simulink model "problem4_simulink_"  (R2021a)
settings: Solver=VariableStepAuto  StartTime=0.0  StopTime=100  RelTol=1e-3
values from neighbouring files (symbols this model uses):
  a4 = init + (last+init)*rand(N,1)    [problem4_code_.m]
  a_hat_ic = init + (last+init)*rand(N,1)    [problem4_code_.m]
  alpha4 = 0.1    [problem4_code_.m]
  beta4 = 0.1    [problem4_code_.m]
  c4 = init + (last+init)*rand(N,1)    [problem4_code_.m]
  g4 = 9.8    [problem4_code_.m]
  gamma4 = diag(gamma)    [problem4_code_.m]
  gamma_a4 = 0.1    [problem4_code_.m]
  k4 = init + (last+init)*rand(N,1)    [problem4_code_.m]
  m4 = init + (last+init)*rand(N,1)    [problem4_code_.m]
  phi4 = init + (last+init)*rand(N,1)    [problem4_code_.m]
  s4 = 0.1    [problem4_code_.m]
  theta = [m4, c4, k4]    [problem4_code_.m]
  theta_hat_ic = [init + (last+init)*rand(N,1), init + (last+init)*rand(N,1), init + (last+init)*rand(N,1)]    [problem4_code_.m]
  u_ic4 = 0    [problem4_code_.m]
  x_ic4 = init + (last+init)*randn(N,1)    [problem4_code_.m]
  xd4 = init + (last+init)*randn(N,1)    [problem4_code_.m]
  xdot_ic4 = 0    [problem4_code_.m]
settings Model: Creator=kaush  LastModifiedBy=kaush
settings DebuggingCC: UnderSpecifiedDimensionMsg=warning

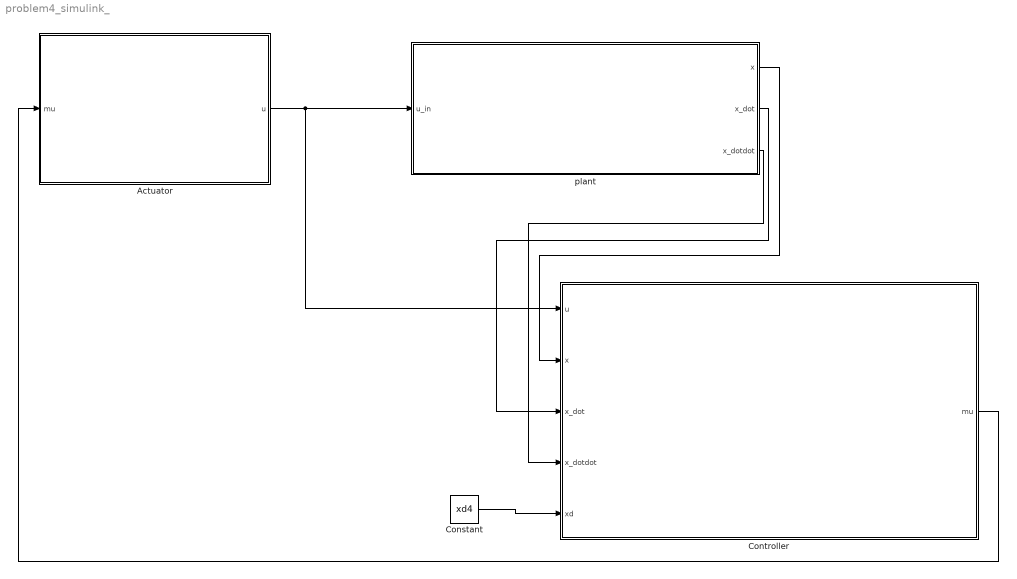
== system problem4_simulink_ ==
  Actuator : Subsystem
  Constant : Constant  Value=xd4
  Controller : Subsystem
  plant : Subsystem
  wires:
  Actuator/1(u) -> Controller/1(u), plant/1(u_in)
  plant/1(x) -> Controller/2(x)
  plant/2(x_dot) -> Controller/3(x_dot)
  plant/3(x_dotdot) -> Controller/4(x_dotdot)
  Constant/1 -> Controller/5(xd)
  Controller/1(mu) -> Actuator/1(mu)

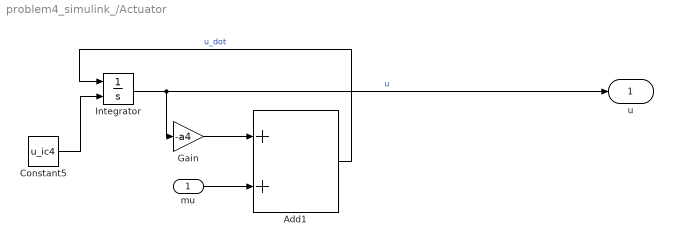
== system problem4_simulink_/Actuator ==
  mu : Inport
  Add1 : Sum
  Constant5 : Constant  Value=u_ic4
  Gain : Gain  Gain=-a4
  Integrator : Integrator  InitialConditionSource=external
  u : Outport
  wires:
  Add1/1 -> Integrator/1  "u_dot"
  Integrator/1 -> u/1, Gain/1  "u"
  Gain/1 -> Add1/1
  mu/1 -> Add1/2
  Constant5/1 -> Integrator/2

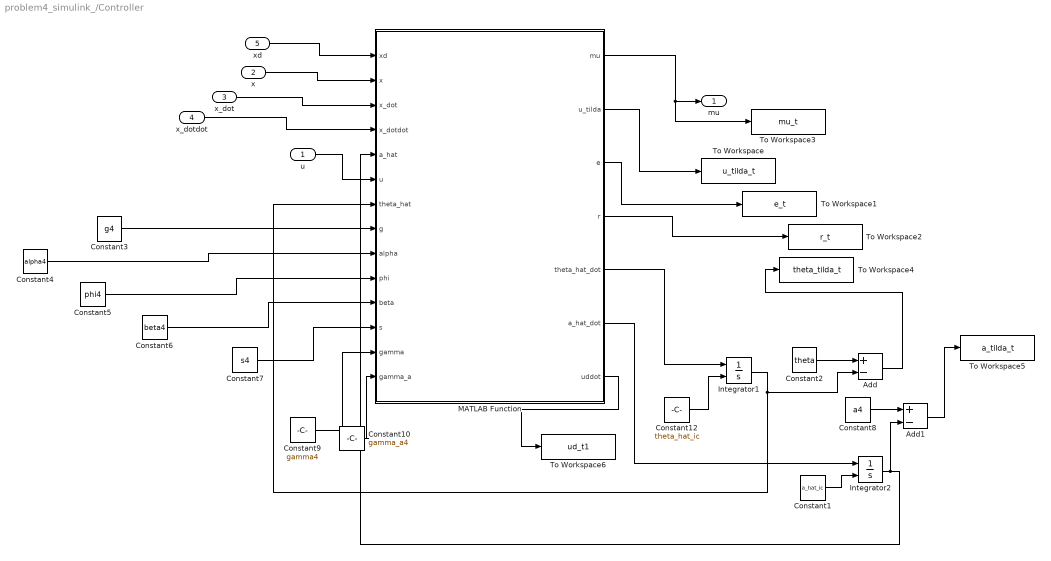
== system problem4_simulink_/Controller ==
  u : Inport
  x : Inport  Port=2
  x_dot : Inport  Port=3
  x_dotdot : Inport  Port=4
  xd : Inport  Port=5
  Add : Sum  Inputs=+-
  Add1 : Sum  Inputs=+-
  Constant1 : Constant  Value=a_hat_ic
  Constant10 : Constant  Value=gamma_a4
  Constant12 : Constant  Value=theta_hat_ic
  Constant2 : Constant  Value=theta
  Constant3 : Constant  Value=g4
  Constant4 : Constant  Value=alpha4
  Constant5 : Constant  Value=phi4
  Constant6 : Constant  Value=beta4
  Constant7 : Constant  Value=s4
  Constant8 : Constant  Value=a4
  Constant9 : Constant  Value=gamma4
  Integrator1 : Integrator  InitialConditionSource=external
  Integrator2 : Integrator  InitialConditionSource=external
  MATLAB Function : MATLAB Function  TreatAsAtomicUnit=on
  To Workspace : ToWorkspace  VariableName=u_tilda_t  SaveFormat=Timeseries  SampleTime=-1
  To Workspace1 : ToWorkspace  VariableName=e_t  SaveFormat=Timeseries  SampleTime=-1
  To Workspace2 : ToWorkspace  VariableName=r_t  SaveFormat=Timeseries  SampleTime=-1
  To Workspace3 : ToWorkspace  VariableName=mu_t  SaveFormat=Timeseries  SampleTime=-1
  To Workspace4 : ToWorkspace  VariableName=theta_tilda_t  SaveFormat=Timeseries  SampleTime=-1
  To Workspace5 : ToWorkspace  VariableName=a_tilda_t  SaveFormat=Timeseries  SampleTime=-1
  To Workspace6 : ToWorkspace  VariableName=ud_t1  SaveFormat=Timeseries  SampleTime=-1
  mu : Outport
  wires:
  x/1 -> MATLAB Function/2(x)
  Constant7/1 -> MATLAB Function/12(s)
  Constant3/1 -> MATLAB Function/8(g)
  Constant6/1 -> MATLAB Function/11(beta)
  Constant4/1 -> MATLAB Function/9(alpha)
  u/1 -> MATLAB Function/6(u)
  x_dotdot/1 -> MATLAB Function/4(x_dotdot)
  xd/1 -> MATLAB Function/1(xd)
  MATLAB Function/3(e) -> To Workspace1/1
  MATLAB Function/2(u_tilda) -> To Workspace/1
  Constant5/1 -> MATLAB Function/10(phi)
  x_dot/1 -> MATLAB Function/3(x_dot)
  MATLAB Function/1(mu) -> To Workspace3/1, mu/1
  MATLAB Function/4(r) -> To Workspace2/1
  Add/1 -> To Workspace4/1
  Add1/1 -> To Workspace5/1
  Constant9/1 -> MATLAB Function/13(gamma)
  Constant10/1 -> MATLAB Function/14(gamma_a)
  Constant12/1 -> Integrator1/2
  MATLAB Function/5(theta_hat_dot) -> Integrator1/1
  Integrator1/1 -> MATLAB Function/7(theta_hat), Add/2
  Constant1/1 -> Integrator2/2
  MATLAB Function/6(a_hat_dot) -> Integrator2/1
  Integrator2/1 -> Add1/2, MATLAB Function/5(a_hat)
  Constant2/1 -> Add/1
  Constant8/1 -> Add1/1
  MATLAB Function/7(uddot) -> To Workspace6/1

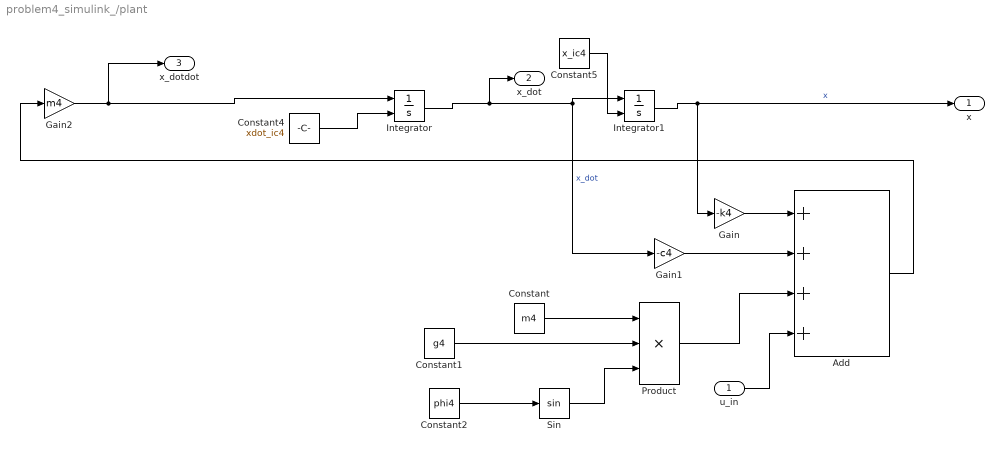
== system problem4_simulink_/plant ==
  u_in : Inport
  Add : Sum  Inputs=++++
  Constant : Constant  Value=m4
  Constant1 : Constant  Value=g4
  Constant2 : Constant  Value=phi4
  Constant4 : Constant  Value=xdot_ic4
  Constant5 : Constant  Value=x_ic4
  Gain : Gain  Gain=-k4
  Gain1 : Gain  Gain=-c4
  Gain2 : Gain  Gain=m4
  Integrator : Integrator  InitialConditionSource=external
  Integrator1 : Integrator  InitialConditionSource=external
  Product : Product  Inputs=3
  Sin : Trigonometry
  x : Outport
  x_dot : Outport  Port=2
  x_dotdot : Outport  Port=3
  wires:
  Constant1/1 -> Product/2
  Product/1 -> Add/3
  Sin/1 -> Product/3
  Constant4/1 -> Integrator/2
  Constant5/1 -> Integrator1/2
  u_in/1 -> Add/4
  Gain2/1 -> Integrator/1, x_dotdot/1
  Integrator/1 -> x_dot/1, Integrator1/1, Gain1/1  "x_dot"
  Gain/1 -> Add/1
  Constant/1 -> Product/1
  Gain1/1 -> Add/2
  Add/1 -> Gain2/1
  Integrator1/1 -> x/1, Gain/1  "x"
  Constant2/1 -> Sin/1

== matlab function problem4_simulink_/Controller/MATLAB Function ==
  data: xd input; mu output; x input; x_dot input; x_dotdot input; a_hat input; u input; theta_hat input; g input; alpha input; phi input; beta input; s input; u_tilda output; e output; r output; gamma input; gamma_a input; theta_hat_dot output; a_hat_dot output; uddot output
function [mu,u_tilda,e,r, theta_hat_dot, a_hat_dot,uddot] = fcn(xd,x,x_dot,x_dotdot, a_hat, u, theta_hat, g, alpha, phi, beta, s, gamma, gamma_a)
e = xd - x;
e_dot = -x_dot;
e_dotdot = -x_dotdot;
r = e_dot + alpha*e;
r_dot = e_dotdot + alpha*e_dot;
Y = [-g*sin(phi)+alpha*e_dot, x_dot, x];
Y_dot = [alpha*e_dotdot, x_dotdot, x_dot];
theta_hat_dot = gamma*Y'*r;
ud = e + beta*r + Y*theta_hat;
u_tilda = ud - u;
a_hat_dot = gamma_a*u_tilda*u;
uddot = Y*theta_hat_dot + Y_dot*theta_hat + e_dot + beta*r_dot;
mu = uddot + a_hat*u + r + s*u_tilda;
